simulink model "PWL_model_Simulink"  (Simulink 9.0)
settings: Solver=ode45  StartTime=0.0  StopTime=T  RelTol=RelTol  AbsTol=AbsTol  EnableMultiTasking=on
values from neighbouring files (symbols this model uses):
  A1 = [-3 1;-5 1]    [PWL_run_Simulink.m]    (also in dwelltimes_bisection.m = [-1 10; -100 -1])
  A2 = [-3 -1;5 1]    [PWL_run_Simulink.m]    (also in dwelltimes_bisection.m = [-1 100; -10 -1])
  x10 = 1    [PWL_run_Simulink.m]
  x20 = 1    [PWL_run_Simulink.m]
settings Model: Creator=drijlaars  LastModifiedBy=ddeenen
settings SolverCC: MaxConsecutiveZCs=1e4
settings DataIOCC: LimitDataPoints=on  SignalLoggingSaveFormat=ModelDataLogs
settings OptimizationCC: ExpressionDepthLimit=2147483647  InitFltsAndDblsToZero=on
settings DebuggingCC: SolverPrmCheckMsg=warning  FcnCallInpInsideContextMsg=warning  StateNameClashWarn=warning  StrictBusMsg=Warning
settings GRTTargetCC: GeneratePreprocessorConditionals=Disable all  CombineOutputUpdateFcns=off  GRTInterface=on

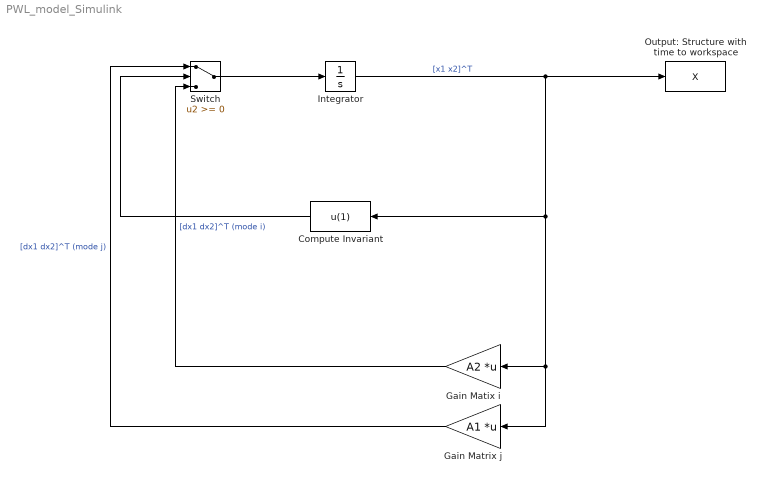
== system PWL_model_Simulink ==
  Compute Invariant : Fcn  Expr=u(1)
  Gain Matix i : Gain  Gain=A2  Multiplication=Matrix(K*u)
  Gain Matrix j : Gain  Gain=A1  Multiplication=Matrix(K*u)
  Integrator : Integrator  InitialCondition=[x10 x20]
  Output: Structure with time to workspace : ToWorkspace  VariableName=X  SaveFormat=Structure With Time  SampleTime=-1
  Switch : Switch
  wires:
  Integrator/1 -> Output: Structure with time to workspace/1, Gain Matix i/1, Gain Matrix j/1, Compute Invariant/1  "[x1 x2]^T"
  Switch/1 -> Integrator/1
  Compute Invariant/1 -> Switch/2
  Gain Matrix j/1 -> Switch/1  "[dx1 dx2]^T (mode j)"
  Gain Matix i/1 -> Switch/3  "[dx1 dx2]^T (mode i)"
